simulink model "PFC_PWM__SCI_Test_3"  (R2021a)
settings: Solver=FixedStepDiscrete  StartTime=0.0  StopTime=Inf  RelTol=1e-3  EnableMultiTasking=on
values from neighbouring files (symbols this model uses):
  AC_V_SENSE_GAIN = 220.2    [PFC_drscrete.m]
  ADC_Gain = 3.3/(2^12)    (= 0.0008056640625)    [PFC_drscrete.m]
  COUNTER_PERIOD = 899    [PFC_drscrete.m]
  DC_BUS_V_GAIN = 307.3830    (= 307.383)    [PFC_drscrete.m]
  Fault_current_Threshold = 100    [PFC_drscrete.m]
  INDUCTOR_1_CURRENT_GAIN = 40    [PFC_drscrete.m]
  INDUCTOR_2_CURRENT_GAIN = 40    [PFC_drscrete.m]
  INDUCTOR_3_CURRENT_GAIN = 40    [PFC_drscrete.m]
  INPUT_AC_CURRENT_GAIN = 1    [PFC_drscrete.m]
  Po = 15000/3    (= 5000)    [PFC_drscrete.m]
  TEMP_SENSE_GAIN = 1    [PFC_drscrete.m]
  TS = 1/1000    (= 0.001)    [PFC_drscrete.m]
  TS_current = 1e-5    (= 1e-05)    [PFC_drscrete.m]
  TS_voltage = 1e-3    (= 0.001)    [PFC_drscrete.m]
  Vm = 400    [PFC_drscrete.m]
undefined symbols (not defined in the file or in its folder): Down, GPTRIP1SEL, GPTRIP2SEL, TZ1, TZ2, Up
libraries: c2802xlib x17, cstblocks x3, c280xlib x2, pid_lib x2
(part 2 of 2)

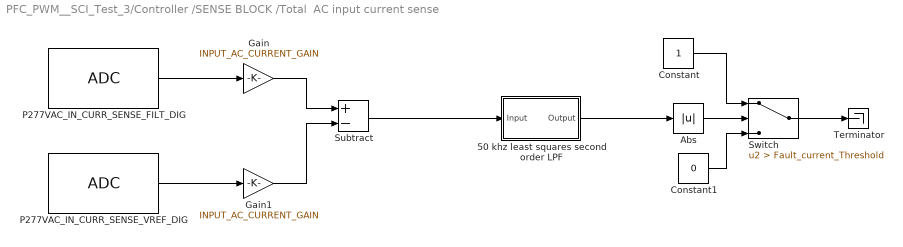
== system PFC_PWM__SCI_Test_3/Controller /SENSE BLOCK /Total  AC input current sense  ==
  50 khz least squares second order LPF : Subsystem  Tag=FilterWizardSubSystem
      settings: ErrorFcn=dspFilterRealizedInBasicElemsAlgLoopErrFcnCallback
  Abs : Abs
  Constant : Constant
  Constant1 : Constant  Value=0
  Gain : Gain  Gain=INPUT_AC_CURRENT_GAIN
  Gain1 : Gain  Gain=INPUT_AC_CURRENT_GAIN
  P277VAC_IN_CURR_SENSE_FILT_DIG : c2802xlib/ADC  blkParamProc=C2000  ADCModule=1  samplingMode=Single sample mode  ADCResolution=12-bit (Single-ended input)  useSOC1=SOC4  useSOC2=SOC0_SOC1  SOCAcquisitionWindow=7  SOCTriggerSource=Software  SOCInterruptTrigger=No ADCINT  Ts=TS  dType=single  postInterrupt=off  interruptSel=ADCINT1  ADCINTContinuous=off  endma=off  chdma=1  conv1=ADCINB7  conv2=ADCINA0 and ADCINB0  conv1_Type4=ADCIN0  conv2_Type4=ADCIN0 and ADCIN1
  P277VAC_IN_CURR_SENSE_VREF_DIG : c2802xlib/ADC  blkParamProc=C2000  ADCModule=1  samplingMode=Single sample mode  ADCResolution=12-bit (Single-ended input)  useSOC1=SOC5  useSOC2=SOC0_SOC1  SOCAcquisitionWindow=7  SOCTriggerSource=Software  SOCInterruptTrigger=No ADCINT  Ts=TS  dType=single  postInterrupt=off  interruptSel=ADCINT1  ADCINTContinuous=off  endma=off  chdma=1  conv1=ADCINA0  conv2=ADCINA0 and ADCINB0  conv1_Type4=ADCIN0  conv2_Type4=ADCIN0 and ADCIN1
  Subtract : Sum  Inputs=+-
  Switch : Switch  Criteria=u2 > Threshold  Threshold=Fault_current_Threshold
  Terminator : Terminator
  wires:
  P277VAC_IN_CURR_SENSE_FILT_DIG/1 -> Gain/1
  Subtract/1 -> 50 khz least squares second order LPF/1(Input)
  Gain1/1 -> Subtract/2
  P277VAC_IN_CURR_SENSE_VREF_DIG/1 -> Gain1/1
  Gain/1 -> Subtract/1
  Abs/1 -> Switch/2
  Constant/1 -> Switch/1
  Constant1/1 -> Switch/3
  Switch/1 -> Terminator/1
  50 khz least squares second order LPF/1(Output) -> Abs/1

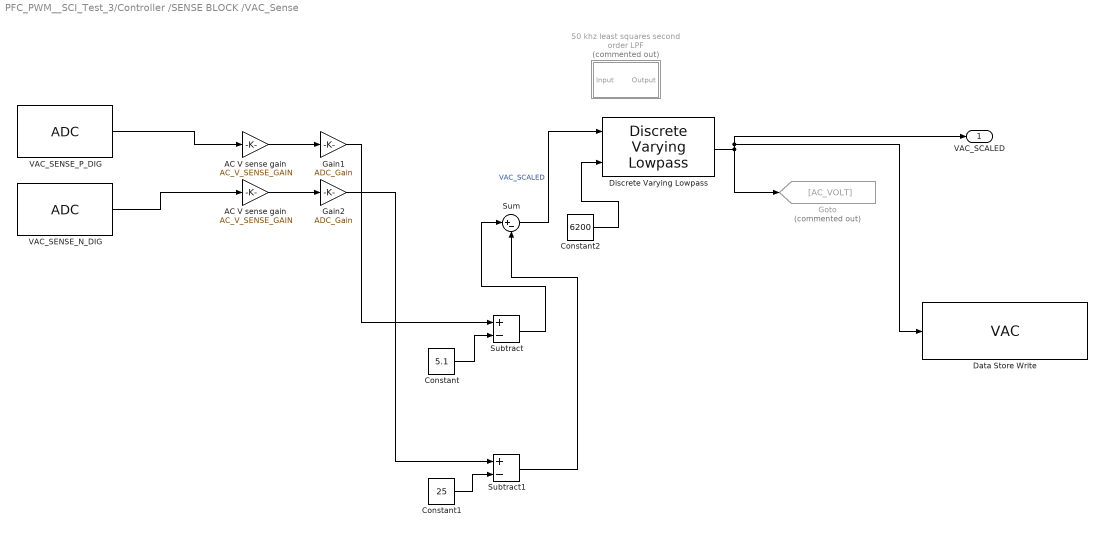
== system PFC_PWM__SCI_Test_3/Controller /SENSE BLOCK /VAC_Sense ==
  50 khz least squares second order LPF : Subsystem  Tag=FilterWizardSubSystem  Commented=on
      settings: ErrorFcn=dspFilterRealizedInBasicElemsAlgLoopErrFcnCallback
  AC V sense gain : Gain  Gain=AC_V_SENSE_GAIN
  "AC V sense gain " : Gain  Gain=AC_V_SENSE_GAIN
  Constant : Constant  Value=5.1
  Constant1 : Constant  Value=25
  Constant2 : Constant  Value=6200
  Data Store Write : DataStoreWrite  DataStoreName=VAC  IndexOptions=Index vector (dialog)  Indices=1  OutputSizes=1
  Discrete Varying Lowpass : cstblocks/Linear Parameter Varying/Discrete Varying Lowpass  N=2  w0=0  Ts=TS_current
      settings: SourceProductBaseCode=CT
  Gain1 : Gain  Gain=ADC_Gain
  Gain2 : Gain  Gain=ADC_Gain
  Goto : Goto  Commented=on  GotoTag=AC_VOLT
  Subtract : Sum  Inputs=+-
  Subtract1 : Sum  Inputs=+-
  Sum : Sum  Inputs=|+-
  VAC_SENSE_N_DIG : c2802xlib/ADC  blkParamProc=C2000  ADCModule=1  samplingMode=Single sample mode  ADCResolution=12-bit (Single-ended input)  useSOC1=SOC1  useSOC2=SOC0_SOC1  SOCAcquisitionWindow=7  SOCTriggerSource=ePWM1_ADCSOCB  SOCInterruptTrigger=No ADCINT  Ts=TS_current  dType=single  postInterrupt=off  interruptSel=ADCINT1  ADCINTContinuous=off  endma=off  chdma=1  conv1=ADCINB1  conv2=ADCINA0 and ADCINB0  conv1_Type4=ADCIN0  conv2_Type4=ADCIN0 and ADCIN1
  VAC_SENSE_P_DIG : c2802xlib/ADC  blkParamProc=C2000  ADCModule=1  samplingMode=Single sample mode  ADCResolution=12-bit (Single-ended input)  useSOC1=SOC0  useSOC2=SOC0_SOC1  SOCAcquisitionWindow=7  SOCTriggerSource=ePWM1_ADCSOCB  SOCInterruptTrigger=No ADCINT  Ts=TS_current  dType=single  postInterrupt=off  interruptSel=ADCINT1  ADCINTContinuous=off  endma=off  chdma=1  conv1=ADCINA7  conv2=ADCINA0 and ADCINB0  conv1_Type4=ADCIN0  conv2_Type4=ADCIN0 and ADCIN1
  VAC_SCALED : Outport  VectorParamsAs1DForOutWhenUnconnected=off
  wires:
  AC V sense gain/1 -> Gain2/1
  Sum/1 -> Discrete Varying Lowpass/1  "VAC_SCALED"
  VAC_SENSE_N_DIG/1 -> AC V sense gain/1
  "AC V sense gain "/1 -> Gain1/1
  Discrete Varying Lowpass/1 -> Data Store Write/1, VAC_SCALED/1, Goto/1
  Constant/1 -> Subtract/2
  Constant1/1 -> Subtract1/2
  Subtract/1 -> Sum/1
  Subtract1/1 -> Sum/2
  VAC_SENSE_P_DIG/1 -> "AC V sense gain "/1
  Gain2/1 -> Subtract1/1
  Gain1/1 -> Subtract/1
  Constant2/1 -> Discrete Varying Lowpass/2

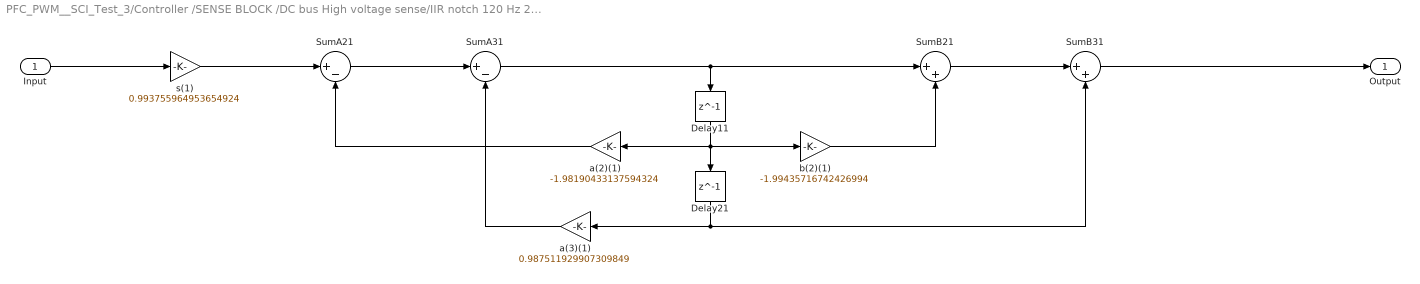
== system PFC_PWM__SCI_Test_3/Controller /SENSE BLOCK /DC bus High voltage sense/IIR notch 120 Hz 2nd order chebyshev  ==
  Input : Inport
  Delay11 : Delay  DelayLength=1  InitialCondition=0
  Delay21 : Delay  DelayLength=1  InitialCondition=0
  SumA21 : Sum  Inputs=|+-  RndMeth=Nearest  SaturateOnIntegerOverflow=on  OutDataTypeStr=Inherit: Same as first input
  SumA31 : Sum  Inputs=|+-  RndMeth=Nearest  SaturateOnIntegerOverflow=on  OutDataTypeStr=Inherit: Same as first input
  SumB21 : Sum  Inputs=|++  RndMeth=Nearest  SaturateOnIntegerOverflow=on  OutDataTypeStr=Inherit: Same as first input
  SumB31 : Sum  Inputs=|++  RndMeth=Nearest  SaturateOnIntegerOverflow=on  OutDataTypeStr=Inherit: Same as first input
  a(2)(1) : Gain  Gain=-1.98190433137594324  ParamDataTypeStr=double  RndMeth=Nearest  SaturateOnIntegerOverflow=on  OutDataTypeStr=Inherit: Same as input
  a(3)(1) : Gain  Gain=0.987511929907309849  ParamDataTypeStr=double  RndMeth=Nearest  SaturateOnIntegerOverflow=on  OutDataTypeStr=Inherit: Same as input
  b(2)(1) : Gain  Gain=-1.99435716742426994  ParamDataTypeStr=double  RndMeth=Nearest  SaturateOnIntegerOverflow=on  OutDataTypeStr=Inherit: Same as input
  s(1) : Gain  Gain=0.993755964953654924  ParamDataTypeStr=double  RndMeth=Nearest  SaturateOnIntegerOverflow=on  OutDataTypeStr=Inherit: Same as input
  Output : Outport
  wires:
  Input/1 -> s(1)/1
  s(1)/1 -> SumA21/1
  SumA21/1 -> SumA31/1
  SumA31/1 -> SumB21/1, Delay11/1
  SumB21/1 -> SumB31/1
  SumB31/1 -> Output/1
  a(2)(1)/1 -> SumA21/2
  Delay11/1 -> a(2)(1)/1, b(2)(1)/1, Delay21/1
  b(2)(1)/1 -> SumB21/2
  a(3)(1)/1 -> SumA31/2
  Delay21/1 -> a(3)(1)/1, SumB31/2

== system PFC_PWM__SCI_Test_3/Controller /SENSE BLOCK /INDUCTOR 1 CURRENT SENSE /50 khz least squares second order LPF ==
  Input : Inport
  BodyDelay2 : Delay  DelayLength=1  InitialCondition=0
  BodyDelay3 : Delay  DelayLength=1  InitialCondition=0
  BodyLSum2 : Sum  Inputs=++|  RndMeth=Nearest  SaturateOnIntegerOverflow=on  OutDataTypeStr=Inherit: Same as first input
  BodyLSum3 : Sum  Inputs=++|  RndMeth=Nearest  SaturateOnIntegerOverflow=on  OutDataTypeStr=Inherit: Same as first input
  b(1) : Gain  Gain=0.311834636224173511  ParamDataTypeStr=double  RndMeth=Nearest  SaturateOnIntegerOverflow=on  OutDataTypeStr=Inherit: Same as input
  b(2) : Gain  Gain=0.544759705509946124  ParamDataTypeStr=double  RndMeth=Nearest  SaturateOnIntegerOverflow=on  OutDataTypeStr=Inherit: Same as input
  b(3) : Gain  Gain=0.311834636224173511  ParamDataTypeStr=double  RndMeth=Nearest  SaturateOnIntegerOverflow=on  OutDataTypeStr=Inherit: Same as input
  Output : Outport
  wires:
  Input/1 -> b(1)/1, BodyDelay2/1
  b(1)/1 -> BodyLSum2/2
  BodyDelay2/1 -> b(2)/1, BodyDelay3/1
  b(2)/1 -> BodyLSum2/1
  BodyLSum2/1 -> BodyLSum3/1
  BodyDelay3/1 -> b(3)/1
  b(3)/1 -> BodyLSum3/2
  BodyLSum3/1 -> Output/1

== system PFC_PWM__SCI_Test_3/Controller /SENSE BLOCK /INDUCTOR 2 CURRENT SENSE /50 khz least squares second order LPF ==
  Input : Inport
  BodyDelay2 : Delay  DelayLength=1  InitialCondition=0
  BodyDelay3 : Delay  DelayLength=1  InitialCondition=0
  BodyLSum2 : Sum  Inputs=++|  RndMeth=Nearest  SaturateOnIntegerOverflow=on  OutDataTypeStr=Inherit: Same as first input
  BodyLSum3 : Sum  Inputs=++|  RndMeth=Nearest  SaturateOnIntegerOverflow=on  OutDataTypeStr=Inherit: Same as first input
  b(1) : Gain  Gain=0.311834636224173511  ParamDataTypeStr=double  RndMeth=Nearest  SaturateOnIntegerOverflow=on  OutDataTypeStr=Inherit: Same as input
  b(2) : Gain  Gain=0.544759705509946124  ParamDataTypeStr=double  RndMeth=Nearest  SaturateOnIntegerOverflow=on  OutDataTypeStr=Inherit: Same as input
  b(3) : Gain  Gain=0.311834636224173511  ParamDataTypeStr=double  RndMeth=Nearest  SaturateOnIntegerOverflow=on  OutDataTypeStr=Inherit: Same as input
  Output : Outport
  wires:
  Input/1 -> b(1)/1, BodyDelay2/1
  b(1)/1 -> BodyLSum2/2
  BodyDelay2/1 -> b(2)/1, BodyDelay3/1
  b(2)/1 -> BodyLSum2/1
  BodyLSum2/1 -> BodyLSum3/1
  BodyDelay3/1 -> b(3)/1
  b(3)/1 -> BodyLSum3/2
  BodyLSum3/1 -> Output/1

== system PFC_PWM__SCI_Test_3/Controller /SENSE BLOCK /INDUCTOR 3 CURRENT SENSE 3/50 khz least squares second order LPF ==
  Input : Inport
  BodyDelay2 : Delay  DelayLength=1  InitialCondition=0
  BodyDelay3 : Delay  DelayLength=1  InitialCondition=0
  BodyLSum2 : Sum  Inputs=++|  RndMeth=Nearest  SaturateOnIntegerOverflow=on  OutDataTypeStr=Inherit: Same as first input
  BodyLSum3 : Sum  Inputs=++|  RndMeth=Nearest  SaturateOnIntegerOverflow=on  OutDataTypeStr=Inherit: Same as first input
  b(1) : Gain  Gain=0.311834636224173511  ParamDataTypeStr=double  RndMeth=Nearest  SaturateOnIntegerOverflow=on  OutDataTypeStr=Inherit: Same as input
  b(2) : Gain  Gain=0.544759705509946124  ParamDataTypeStr=double  RndMeth=Nearest  SaturateOnIntegerOverflow=on  OutDataTypeStr=Inherit: Same as input
  b(3) : Gain  Gain=0.311834636224173511  ParamDataTypeStr=double  RndMeth=Nearest  SaturateOnIntegerOverflow=on  OutDataTypeStr=Inherit: Same as input
  Output : Outport
  wires:
  Input/1 -> b(1)/1, BodyDelay2/1
  b(1)/1 -> BodyLSum2/2
  BodyDelay2/1 -> b(2)/1, BodyDelay3/1
  b(2)/1 -> BodyLSum2/1
  BodyLSum2/1 -> BodyLSum3/1
  BodyDelay3/1 -> b(3)/1
  b(3)/1 -> BodyLSum3/2
  BodyLSum3/1 -> Output/1

== system PFC_PWM__SCI_Test_3/Controller /SENSE BLOCK /Power stage temperature sense /1 khz least squares second order LPF ==
  Input : Inport
  BodyDelay2 : Delay  DelayLength=1  InitialCondition=0
  BodyDelay3 : Delay  DelayLength=1  InitialCondition=0
  BodyLSum2 : Sum  Inputs=++|  RndMeth=Nearest  SaturateOnIntegerOverflow=on  OutDataTypeStr=Inherit: Same as first input
  BodyLSum3 : Sum  Inputs=++|  RndMeth=Nearest  SaturateOnIntegerOverflow=on  OutDataTypeStr=Inherit: Same as first input
  b(1) : Gain  Gain=0.306687619047849525  ParamDataTypeStr=double  RndMeth=Nearest  SaturateOnIntegerOverflow=on  OutDataTypeStr=Inherit: Same as input
  b(2) : Gain  Gain=0.499999999999999889  ParamDataTypeStr=double  RndMeth=Nearest  SaturateOnIntegerOverflow=on  OutDataTypeStr=Inherit: Same as input
  b(3) : Gain  Gain=0.306687619047849525  ParamDataTypeStr=double  RndMeth=Nearest  SaturateOnIntegerOverflow=on  OutDataTypeStr=Inherit: Same as input
  Output : Outport
  wires:
  Input/1 -> b(1)/1, BodyDelay2/1
  b(1)/1 -> BodyLSum2/2
  BodyDelay2/1 -> b(2)/1, BodyDelay3/1
  b(2)/1 -> BodyLSum2/1
  BodyLSum2/1 -> BodyLSum3/1
  BodyDelay3/1 -> b(3)/1
  b(3)/1 -> BodyLSum3/2
  BodyLSum3/1 -> Output/1

== system PFC_PWM__SCI_Test_3/Controller /SENSE BLOCK /Total  AC input current sense /50 khz least squares second order LPF ==
  Input : Inport
  BodyDelay2 : Delay  DelayLength=1  InitialCondition=0
  BodyDelay3 : Delay  DelayLength=1  InitialCondition=0
  BodyLSum2 : Sum  Inputs=++|  RndMeth=Nearest  SaturateOnIntegerOverflow=on  OutDataTypeStr=Inherit: Same as first input
  BodyLSum3 : Sum  Inputs=++|  RndMeth=Nearest  SaturateOnIntegerOverflow=on  OutDataTypeStr=Inherit: Same as first input
  b(1) : Gain  Gain=0.311834636224173511  ParamDataTypeStr=double  RndMeth=Nearest  SaturateOnIntegerOverflow=on  OutDataTypeStr=Inherit: Same as input
  b(2) : Gain  Gain=0.544759705509946124  ParamDataTypeStr=double  RndMeth=Nearest  SaturateOnIntegerOverflow=on  OutDataTypeStr=Inherit: Same as input
  b(3) : Gain  Gain=0.311834636224173511  ParamDataTypeStr=double  RndMeth=Nearest  SaturateOnIntegerOverflow=on  OutDataTypeStr=Inherit: Same as input
  Output : Outport
  wires:
  Input/1 -> b(1)/1, BodyDelay2/1
  b(1)/1 -> BodyLSum2/2
  BodyDelay2/1 -> b(2)/1, BodyDelay3/1
  b(2)/1 -> BodyLSum2/1
  BodyLSum2/1 -> BodyLSum3/1
  BodyDelay3/1 -> b(3)/1
  b(3)/1 -> BodyLSum3/2
  BodyLSum3/1 -> Output/1

== system PFC_PWM__SCI_Test_3/Controller /SENSE BLOCK /VAC_Sense/50 khz least squares second order LPF ==
  Input : Inport
  BodyDelay2 : Delay  DelayLength=1  InitialCondition=0
  BodyDelay3 : Delay  DelayLength=1  InitialCondition=0
  BodyLSum2 : Sum  Inputs=++|  RndMeth=Nearest  SaturateOnIntegerOverflow=on  OutDataTypeStr=Inherit: Same as first input
  BodyLSum3 : Sum  Inputs=++|  RndMeth=Nearest  SaturateOnIntegerOverflow=on  OutDataTypeStr=Inherit: Same as first input
  b(1) : Gain  Gain=0.311834636224173511  ParamDataTypeStr=double  RndMeth=Nearest  SaturateOnIntegerOverflow=on  OutDataTypeStr=Inherit: Same as input
  b(2) : Gain  Gain=0.544759705509946124  ParamDataTypeStr=double  RndMeth=Nearest  SaturateOnIntegerOverflow=on  OutDataTypeStr=Inherit: Same as input
  b(3) : Gain  Gain=0.311834636224173511  ParamDataTypeStr=double  RndMeth=Nearest  SaturateOnIntegerOverflow=on  OutDataTypeStr=Inherit: Same as input
  Output : Outport
  wires:
  Input/1 -> b(1)/1, BodyDelay2/1
  b(1)/1 -> BodyLSum2/2
  BodyDelay2/1 -> b(2)/1, BodyDelay3/1
  b(2)/1 -> BodyLSum2/1
  BodyLSum2/1 -> BodyLSum3/1
  BodyDelay3/1 -> b(3)/1
  b(3)/1 -> BodyLSum3/2
  BodyLSum3/1 -> Output/1
